simulink model "task_01_1_2"  (R2021b)
settings: Solver=VariableStepAuto  StartTime=0.0  StopTime=10.0  RelTol=1e-3
settings Model: Creator=User_Admin  LastModifiedBy=User_Admin

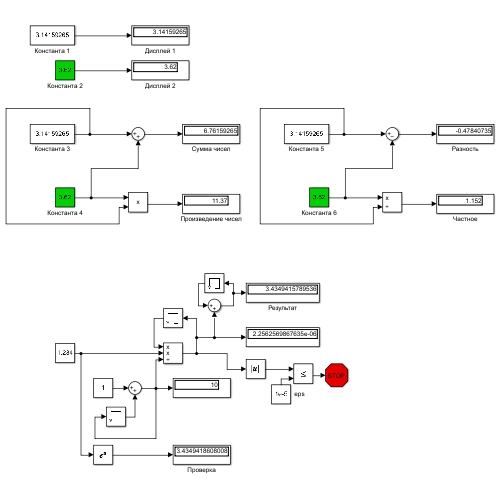
[thumbnail: Simulink's stored preview of the top-level diagram]
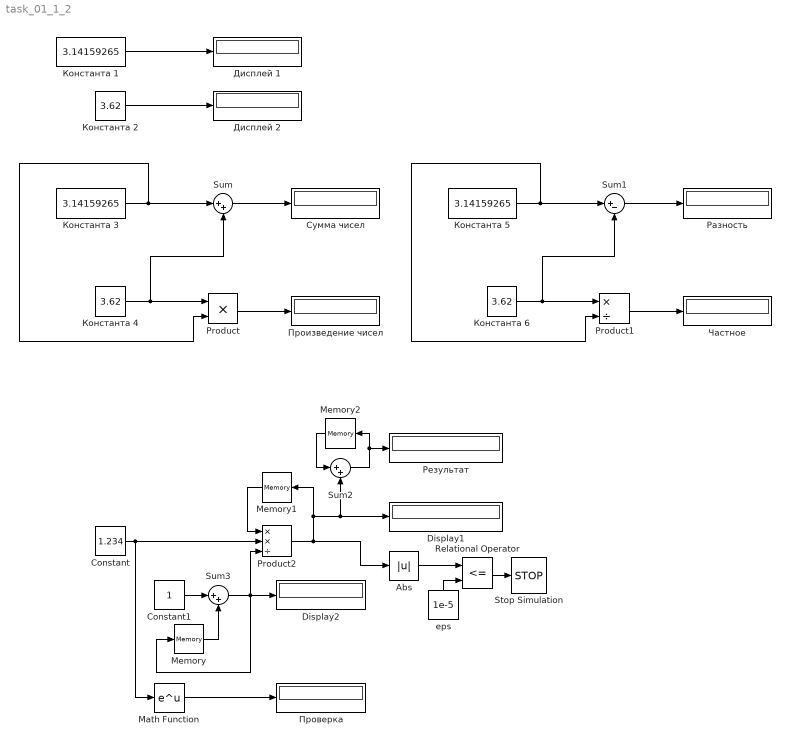
== system task_01_1_2 ==
  Abs : Abs
  Constant : Constant  Value=1.234
  Constant1 : Constant
  Display1 : Display
  Display2 : Display
  Math Function : Math  SaturateOnIntegerOverflow=on
  Memory : Memory
  Memory1 : Memory  InitialCondition=1
  Memory2 : Memory  InitialCondition=1
  Product : Product
  Product1 : Product  Inputs=*/
  Product2 : Product  Inputs=**/
  Relational Operator : RelationalOperator  Operator=<=  OutDataTypeStr=boolean  RndMeth=Simplest
  Stop Simulation : Stop
  Sum : Sum  Inputs=|++
  Sum1 : Sum  Inputs=|+-
  Sum2 : Sum  Inputs=|++
  Sum3 : Sum  Inputs=|++
  eps : Constant  Value=1e-5
  Дисплей 1 : Display
  Дисплей 2 : Display
  Константа 1 : Constant  Value=3.14159265
  Константа 2 : Constant  Value=3.62
  Константа 3 : Constant  Value=3.14159265
  Константа 4 : Constant  Value=3.62
  Константа 5 : Constant  Value=3.14159265
  Константа 6 : Constant  Value=3.62
  Проверка : Display
  Произведение чисел : Display
  Разность : Display
  Результат : Display
  Сумма чисел : Display
  Частное : Display
  wires:
  Product/1 -> Произведение чисел/1
  Sum/1 -> Сумма чисел/1
  Константа 4/1 -> Product/1, Sum/2
  Константа 3/1 -> Sum/1, Product/2
  Константа 1/1 -> Дисплей 1/1
  Константа 2/1 -> Дисплей 2/1
  Sum1/1 -> Разность/1
  Константа 6/1 -> Product1/1, Sum1/2
  Константа 5/1 -> Sum1/1, Product1/2
  Product1/1 -> Частное/1
  eps/1 -> Relational Operator/2
  Abs/1 -> Relational Operator/1
  Product2/1 -> Sum2/2, Display1/1, Memory1/1, Abs/1
  Sum3/1 -> Product2/3, Memory/1, Display2/1
  Memory/1 -> Sum3/2
  Constant1/1 -> Sum3/1
  Constant/1 -> Product2/2, Math Function/1
  Math Function/1 -> Проверка/1
  Memory1/1 -> Product2/1
  Relational Operator/1 -> Stop Simulation/1
  Sum2/1 -> Memory2/1, Результат/1
  Memory2/1 -> Sum2/1
